simulink model "UFR_Controller"  (R2023a)
settings: Solver=FixedStepDiscrete  StartTime=0.0  StopTime=10  FixedStep=0.01  RelTol=1e-3
undefined symbols (not defined in the file): out
settings Model: PacingRate=0.100000  Creator=alibacon  LastModifiedBy=ppatel
settings DataIOCC: SaveOutput=off  SaveTime=off
settings OptimizationCC: BlockReduction=off  DefaultParameterBehavior=Inlined  UseDivisionForNetSlopeComputation=on  GainParamInheritBuiltInType=on  UseFloatMulNetSlope=on  InlineInvariantSignals=on  PassReuseOutputArgsAs=Individual arguments  EfficientFloat2IntCast=on  LifeSpan=inf  OptimizeBlockOrder=speed  DifferentSizesBufferReuse=on  EfficientTunableParamExpr=on
settings DebuggingCC: SignalInfNanChecking=error  SignalRangeChecking=error  ReadBeforeWriteMsg=EnableAllAsError  WriteAfterWriteMsg=EnableAllAsError  WriteAfterReadMsg=EnableAllAsError  AlgebraicLoopMsg=error  ArtificialAlgebraicLoopMsg=error  SaveWithDisabledLinksMsg=error  SaveWithParameterizedLinksMsg=error  BlockPriorityViolationMsg=error  SolverPrmCheckMsg=error  InheritedTsInSrcMsg=error  SingleTaskRateTransMsg=error  TasksWithSamePriorityMsg=error  SigSpecEnsureSampleTimeMsg=error  CheckMatrixSingularityMsg=error  IntegerOverflowMsg=error  ParameterUnderflowMsg=error  ParameterPrecisionLossMsg=error  ParameterTunabilityLossMsg=error  UnderSpecifiedDataTypeMsg=error  UnnecessaryDatatypeConvMsg=warning  VectorMatrixConversionMsg=error  SignalLabelMismatchMsg=error  UnconnectedInputMsg=error  UnconnectedOutputMsg=error  UnconnectedLineMsg=error  SFcnCompatibilityMsg=error  UniqueDataStoreMsg=error  BusObjectLabelMismatch=error  RootOutportRequireBusObject=error  AssertControl=DisableAll  ModelReferenceIOMsg=error  ModelReferenceIOMismatchMessage=error  UnknownTsInhSupMsg=error  ModelReferenceDataLoggingMessage=error  StateNameClashWarn=warning  SubsystemReferenceDiagnosticForUnitTest=warning  StrictBusMsg=ErrorOnBusTreatedAsVector  NonBusSignalsTreatedAsBus=error  SFInvalidInputDataAccessInChartInitDiag=error  SFTransitionOutsideNaturalParentDiag=error  SFUnreachableExecutionPathDiag=error  SFUndirectedBroadcastEventsDiag=error  SFTransitionActionBeforeConditionDiag=error  SFTemporalDelaySmallerThanSampleTimeDiag=error  SFSelfTransitionDiag=error  SFExecutionAtInitializationDiag=error  IntegerSaturationMsg=error  VariantConditionMismatch=error
settings HardwareCC: ProdBitPerPointer=32  ProdBitPerSizeT=32  ProdBitPerPtrDiffT=32  ProdLargestAtomicInteger=Long  ProdWordSize=32  ProdLongLongMode=on  ProdHWDeviceType=ARM Compatible->ARM 10
settings SFSimCC: CompileTimeRecursionLimit=0  EnableRuntimeRecursion=off  MATLABDynamicMemAlloc=off
settings RTWCC: Description=Embedded Coder  SystemTargetFile=ert.tlc  TemplateMakefile=ert_default_tmf  GenerateReport=on  LaunchReport=on
settings CodeAppCC: ForceParamTrailComments=on  IgnoreCustomStorageClasses=off  OperatorAnnotations=on  SimulinkDataObjDesc=on  SFDataObjDesc=on  MATLABFcnDesc=on  MangleLength=4  CustomSymbolStrGlobalVar=rt$N$M  CustomSymbolStrType=$N$M  CustomSymbolStrFcn=$N$M$F  CustomSymbolStrMacro=$N$M  InsertBlockDesc=on  ReqsInCode=on
settings ERTTargetCC: TargetLangStandard=C99 (ISO)  UtilityFuncGeneration=Shared location  GenerateSampleERTMain=on  IncludeMdlTerminateFcn=off  CombineSignalStateStructs=on  SuppressErrorStatus=on  SupportAbsoluteTime=off  SupportNonFinite=off  SupportComplex=off  ParenthesesLevel=Standards  CastingMode=Standards  InlinedParameterPlacement=NonHierarchical  ERTCustomFileTemplate=example_file_process.tlc  ERTFilePackagingFormat=CompactWithDataFile  PreserveExpressionOrder=on  SuppressUnreachableDefaultCases=off  EnableSignedLeftShifts=off  EnableSignedRightShifts=off
settings ConfigComp: DVMode=DesignErrorDetection  DVTestSuiteOptimization=Auto  DVDetectDeadLogic=on  DVDetectActiveLogic=on  DVDetectOutOfBounds=on  DVModelReferenceHarness=on  DVHarnessSource=Signal Editor

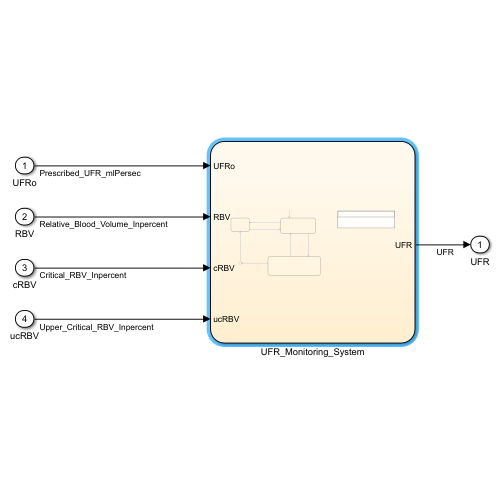
[thumbnail: Simulink's stored preview of the top-level diagram]
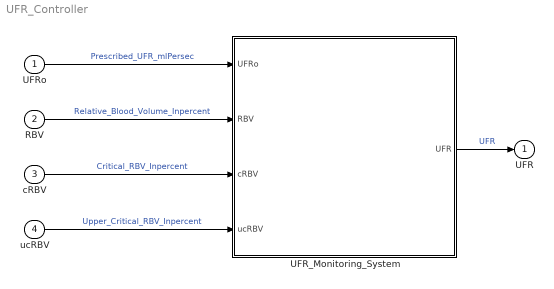
== system UFR_Controller ==
  UFRo : Inport  OutMin=0  OutMax=255  OutDataTypeStr=double  PortDimensions=1  SampleTime=0.01
  RBV : Inport  Port=2  OutMin=0  OutMax=255  OutDataTypeStr=double  PortDimensions=1  SampleTime=0.01
  cRBV : Inport  Port=3  OutMin=0  OutMax=255  OutDataTypeStr=double  PortDimensions=1  SampleTime=0.01
  ucRBV : Inport  Port=4  OutMin=0  OutMax=255  OutDataTypeStr=double  PortDimensions=1  SampleTime=0.01
  UFR_Monitoring_System : Stateflow chart  TreatAsAtomicUnit=on
  UFR : Outport  OutMin=0  OutMax=255  OutDataTypeStr=double  PortDimensions=1  SampleTime=[0,1]
  wires:
  UFRo/1 -> UFR_Monitoring_System/1(UFRo)  "Prescribed_UFR_mlPersec"
  RBV/1 -> UFR_Monitoring_System/2(RBV)  "Relative_Blood_Volume_Inpercent"
  cRBV/1 -> UFR_Monitoring_System/3(cRBV)  "Critical_RBV_Inpercent"
  ucRBV/1 -> UFR_Monitoring_System/4(ucRBV)  "Upper_Critical_RBV_Inpercent"
  UFR_Monitoring_System/1(UFR) -> UFR/1  "UFR"

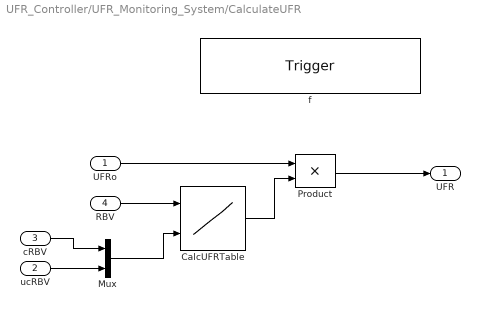
== system UFR_Controller/UFR_Monitoring_System/CalculateUFR ==
  UFRo : Inport  OutDataTypeStr=double  PortDimensions=1
  ucRBV : Inport  Port=2  OutDataTypeStr=double  PortDimensions=1
  cRBV : Inport  Port=3  OutDataTypeStr=double  PortDimensions=1
  RBV : Inport  Port=4  OutDataTypeStr=double  PortDimensions=1
  f : TriggerPort  TriggerType=function-call  VariantControl=(inherit)
      settings: CopyFcn=Stateflow.SLINSF.SimulinkMan.removeBlockPreDeleteFcn  PreDeleteFcn=Stateflow.SLINSF.SimulinkMan.unsafePredeleteFcn
  CalcUFRTable : Lookup_n-D  NumberOfTableDimensions=1  BreakpointsForDimension1Source=Input port  BreakpointsForDimension1=[out.cRBV out.ucRBV]  Table=[0 1]  InternalRulePriority=Speed  RndMeth=Simplest
      settings: InputPortMap=u0,p5
  Mux : Mux  Inputs=2
  Product : Product
  UFR : Outport
  wires:
  RBV/1 -> CalcUFRTable/1
  cRBV/1 -> Mux/1
  UFRo/1 -> Product/1
  Mux/1 -> CalcUFRTable/2
  ucRBV/1 -> Mux/2
  CalcUFRTable/1 -> Product/2
  Product/1 -> UFR/1

== stateflow chart UFR_Controller/UFR_Monitoring_System ==
  state UFR = CalculateUFR(UFRo,ucRBV,cRBV,RBV) [function]
  state Stop
    UFR= double(0);
  state NoCalc
    UFR=UFRo;
  state ReCalc
    UFR = CalculateUFR(UFRo,ucRBV,cRBV,RBV);
  (default) -> NoCalc
  NoCalc -> Stop [order 2] : [RBV <= cRBV]
  Stop -> NoCalc : [RBV > cRBV]
  (junction 68) -> Stop
  ReCalc -> NoCalc [order 1] : [RBV >= ucRBV]
  NoCalc -> ReCalc [order 1] : [(RBV > cRBV) && (RBV < ucRBV)]
  ReCalc -> (junction 68) [order 2] : [RBV <= cRBV]
  data: UFRo function_input double size=1; ucRBV function_input double size=1; cRBV function_input double size=1; RBV function_input double size=1; UFR function_output; UFRo input; RBV input; cRBV input; UFR output; ucRBV input
